simulink model "CAN_T_R_Model"  (R2018a)
settings: Solver=VariableStepAuto  StartTime=0.0  StopTime=10  RelTol=1e-3
undefined symbols (not defined in the file): canChannel
libraries: simulink x16, canlib x5, canmsglib x3
settings Model: Creator=arthu  LastModifiedBy=arthu

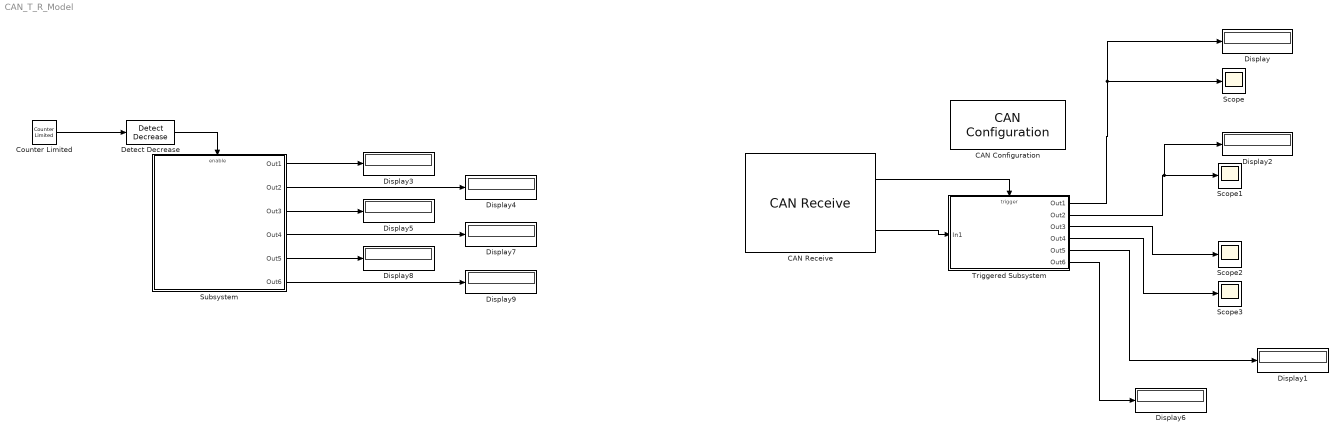
== system CAN_T_R_Model ==
  CAN Configuration : canlib/CAN Configuration  BlockHandle=2149.0007  DeviceMenu=(none)  Device=PEAK-System PCAN-USB (PCAN_USBBUS2)  ObjConstructor=canChannel('MathWorks','Virtual 1',1)  BusSpeed=1000000  EnableBitParameters=off  AckMode=Normal
      settings: SourceProductName=Vehicle Network Toolbox  SourceProductBaseCode=VN
  CAN Receive : canlib/CAN Receive  BlockHandle=2001.0005  DeviceMenu=(none)  Device=PEAK-System PCAN-USB (PCAN_USBBUS2)  ObjConstructor=canChannel('PEAK-System','PCAN_USBBUS1')  EnableStandardIDsFilter=off  StandardIDs=0  EnableExtendedIDsFilter=off  ExtendedIDs=0  SampleTime=0.001  MsgsPerTimestep=all  StdIDsCombo=Allow all  ExtIDsCombo=Allow all  InternalFilterUpdateStatus=on  BusOutput=off
      settings: SourceProductName=Vehicle Network Toolbox  SourceProductBaseCode=VN
  Counter Limited : simulink/Sources/Counter Limited  uplimit=24  tsamp=0.001
  Detect Decrease : simulink/Logic and Bit Operations/Detect Decrease  vinit=0.0  OutDataTypeStr=boolean
  Display{,1..9} (10 alike) : Display
  Scope{,1..3} (4 alike) : Scope
  Subsystem : Subsystem
  Triggered Subsystem : Subsystem  TreatAsAtomicUnit=on
  wires:
  Detect Decrease/1 -> Subsystem/Enable
  Counter Limited/1 -> Detect Decrease/1
  CAN Receive/2 -> Triggered Subsystem/1(In1)
  CAN Receive/1 -> Triggered Subsystem/Trigger
  Triggered Subsystem/1(Out1) -> Display/1, Scope/1
  Triggered Subsystem/2(Out2) -> Display2/1, Scope1/1
  Triggered Subsystem/3(Out3) -> Scope2/1
  Triggered Subsystem/4(Out4) -> Scope3/1
  Triggered Subsystem/5(Out5) -> Display1/1
  Subsystem/1(Out1) -> Display3/1
  Subsystem/2(Out2) -> Display4/1
  Subsystem/3(Out3) -> Display5/1
  Triggered Subsystem/6(Out6) -> Display6/1
  Subsystem/4(Out4) -> Display7/1
  Subsystem/6(Out6) -> Display9/1
  Subsystem/5(Out5) -> Display8/1

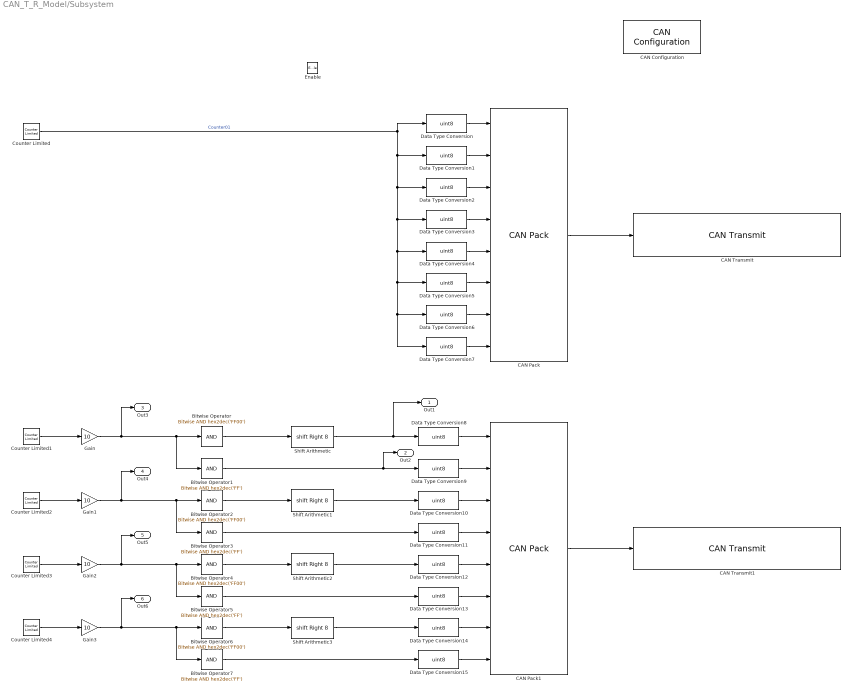
== system CAN_T_R_Model/Subsystem ==
  Enable : EnablePort
  Bitwise Operator{,2,4,6} (4 alike) : simulink/Logic and Bit Operations/Bitwise Operator  logicop=AND  UseBitMask=on  BitMask=hex2dec('FF00')  BitMaskRealWorld=Stored Integer
  Bitwise Operator{1,3,5,7} (4 alike) : simulink/Logic and Bit Operations/Bitwise Operator  logicop=AND  UseBitMask=on  BitMask=hex2dec('FF')  BitMaskRealWorld=Stored Integer
  CAN Configuration : canlib/CAN Configuration  BlockHandle=17.0002  DeviceMenu=PEAK-System PCAN-USB (PCAN_USBBUS1)  Device=PEAK-System PCAN-USB (PCAN_USBBUS1)  ObjConstructor=canChannel('PEAK-System','PCAN_USBBUS1')  BusSpeed=1000000  EnableBitParameters=off  AckMode=Normal
      settings: SourceProductName=Vehicle Network Toolbox  SourceProductBaseCode=VN
  CAN Pack : canmsglib/CAN Pack  MsgList=(none)  MsgName=CAN Msg  MsgIDType=Extended (29-bit identifier)  MsgIdentifier=2000  MsgLength=8  SignalInfo=Signal1$0$8$1$2$1$0$1$0$-Inf$Inf$#Signal2$8$8$1$2$1$0$1$0$-Inf$Inf$#Signal3$16$8$1$2$1$0$1$0$-Inf$Inf$#Signal4$24$8$1$2$1$0$1$0$-Inf$Inf$#Signal5$32$8$1$2$1$0$1$0$-Inf$Inf$#Signal6$40$8$1$2$1$0$1$0$-Inf$Inf$#Signal7$48$8$1$2$1$0$1$0$-Inf$Inf$#Signal8$56$8$1$2$1$0$1$0$-Inf$Inf$#  NSignals=8  StartBits=str2num('[int32(0);int32(8);int32(16);int32(24);int32(32);int32(40);int32(48);int32(56)]')  SignalSizes=str2num('[int32(8);int32(8);int32(8);int32(8);int32(8);int32(8);int32(8);int32(8)]')  ByteOrders=str2num('[int32(1);int32(1);int32(1);int32(1);int32(1);int32(1);int32(1);int32(1)]')  DataTypes=str2num('[int32(2);int32(2);int32(2);int32(2);int32(2);int32(2);int32(2);int32(2)]')  MultiplexTypes=str2num('[int32(1);int32(1);int32(1);int32(1);int32(1);int32(1);int32(1);int32(1)]')  MultiplexValues=str2num('[double(0);double(0);double(0);double(0);double(0);double(0);double(0);double(0)]')  Factors=str2num('[double(1);double(1);double(1);double(1);double(1);double(1);double(1);double(1)]')  Offsets=str2num('[double(0);double(0);double(0);double(0);double(0);double(0);double(0);double(0)]')  Minimums=str2num('[double(-Inf);double(-Inf);double(-Inf);double(-Inf);double(-Inf);double(-Inf);double(-Inf);double(-Inf)]')  Maximums=str2num('[double(Inf);double(Inf);double(Inf);double(Inf);double(Inf);double(Inf);double(Inf);double(Inf)]')  Remote=off  ApplyMinMax=off  BusOutput=off
      settings: SourceProductName=Simulink Real-Time  SourceProductBaseCode=XP  DataFormat=manually specified signals
  CAN Pack1 : canmsglib/CAN Pack  MsgList=(none)  MsgName=CAN Msg  MsgIDType=Extended (29-bit identifier)  MsgIdentifier=2001  MsgLength=8  SignalInfo=Signal1$0$8$1$2$1$0$1$0$-Inf$Inf$#Signal2$8$8$1$2$1$0$1$0$-Inf$Inf$#Signal3$16$8$1$2$1$0$1$0$-Inf$Inf$#Signal4$24$8$1$2$1$0$1$0$-Inf$Inf$#Signal5$32$8$1$2$1$0$1$0$-Inf$Inf$#Signal6$40$8$1$2$1$0$1$0$-Inf$Inf$#Signal7$48$8$1$2$1$0$1$0$-Inf$Inf$#Signal8$56$8$1$2$1$0$1$0$-Inf$Inf$#  NSignals=8  StartBits=str2num('[int32(0);int32(8);int32(16);int32(24);int32(32);int32(40);int32(48);int32(56)]')  SignalSizes=str2num('[int32(8);int32(8);int32(8);int32(8);int32(8);int32(8);int32(8);int32(8)]')  ByteOrders=str2num('[int32(1);int32(1);int32(1);int32(1);int32(1);int32(1);int32(1);int32(1)]')  DataTypes=str2num('[int32(2);int32(2);int32(2);int32(2);int32(2);int32(2);int32(2);int32(2)]')  MultiplexTypes=str2num('[int32(1);int32(1);int32(1);int32(1);int32(1);int32(1);int32(1);int32(1)]')  MultiplexValues=str2num('[double(0);double(0);double(0);double(0);double(0);double(0);double(0);double(0)]')  Factors=str2num('[double(1);double(1);double(1);double(1);double(1);double(1);double(1);double(1)]')  Offsets=str2num('[double(0);double(0);double(0);double(0);double(0);double(0);double(0);double(0)]')  Minimums=str2num('[double(-Inf);double(-Inf);double(-Inf);double(-Inf);double(-Inf);double(-Inf);double(-Inf);double(-Inf)]')  Maximums=str2num('[double(Inf);double(Inf);double(Inf);double(Inf);double(Inf);double(Inf);double(Inf);double(Inf)]')  Remote=off  ApplyMinMax=off  BusOutput=off
      settings: SourceProductName=Simulink Real-Time  SourceProductBaseCode=XP  DataFormat=manually specified signals
  CAN Transmit : canlib/CAN Transmit  BlockHandle=15.0001  DeviceMenu=PEAK-System PCAN-USB (PCAN_USBBUS1)  Device=PEAK-System PCAN-USB (PCAN_USBBUS1)  ObjConstructor=canChannel('PEAK-System','PCAN_USBBUS1')  EnablePeriodicTransmit=off  MessagePeriod=0.050
      settings: SourceProductName=Vehicle Network Toolbox  SourceProductBaseCode=VN
  CAN Transmit1 : canlib/CAN Transmit  BlockHandle=2090.0005  DeviceMenu=PEAK-System PCAN-USB (PCAN_USBBUS1)  Device=PEAK-System PCAN-USB (PCAN_USBBUS1)  ObjConstructor=canChannel('PEAK-System','PCAN_USBBUS1')  EnablePeriodicTransmit=off  MessagePeriod=0.050
      settings: SourceProductName=Vehicle Network Toolbox  SourceProductBaseCode=VN
  Counter Limited{,1..4} (5 alike) : simulink/Sources/Counter Limited  uplimit=255  tsamp=-1
  Data Type Conversion{,1..15} (16 alike) : DataTypeConversion  OutDataTypeStr=uint8
  Gain{,1..3} (4 alike) : Gain  Gain=10  OutDataTypeStr=uint16
  Shift Arithmetic{,1..3} (4 alike) : ArithShift  BitShiftNumber=8  BitShiftDirection=Right
  Out1 : Outport
  Out2 : Outport  Port=2
  Out3 : Outport  Port=3
  Out4 : Outport  Port=4
  Out5 : Outport  Port=5
  Out6 : Outport  Port=6
  wires:
  Data Type Conversion1/1 -> CAN Pack/2
  Data Type Conversion3/1 -> CAN Pack/4
  CAN Pack/1 -> CAN Transmit/1
  Data Type Conversion2/1 -> CAN Pack/3
  Data Type Conversion6/1 -> CAN Pack/7
  Data Type Conversion/1 -> CAN Pack/1
  Data Type Conversion5/1 -> CAN Pack/6
  Data Type Conversion7/1 -> CAN Pack/8
  Data Type Conversion4/1 -> CAN Pack/5
  CAN Pack1/1 -> CAN Transmit1/1
  Counter Limited/1 -> Data Type Conversion/1, Data Type Conversion6/1, Data Type Conversion7/1, Data Type Conversion5/1, Data Type Conversion4/1, Data Type Conversion3/1, Data Type Conversion2/1, Data Type Conversion1/1  "Counter01"
  Data Type Conversion8/1 -> CAN Pack1/1
  Data Type Conversion9/1 -> CAN Pack1/2
  Data Type Conversion10/1 -> CAN Pack1/3
  Data Type Conversion11/1 -> CAN Pack1/4
  Data Type Conversion12/1 -> CAN Pack1/5
  Data Type Conversion13/1 -> CAN Pack1/6
  Data Type Conversion14/1 -> CAN Pack1/7
  Data Type Conversion15/1 -> CAN Pack1/8
  Bitwise Operator/1 -> Shift Arithmetic/1
  Bitwise Operator1/1 -> Out2/1, Data Type Conversion9/1
  Shift Arithmetic/1 -> Out1/1, Data Type Conversion8/1
  Bitwise Operator3/1 -> Data Type Conversion11/1
  Bitwise Operator2/1 -> Shift Arithmetic1/1
  Shift Arithmetic1/1 -> Data Type Conversion10/1
  Bitwise Operator4/1 -> Shift Arithmetic2/1
  Bitwise Operator5/1 -> Data Type Conversion13/1
  Shift Arithmetic2/1 -> Data Type Conversion12/1
  Bitwise Operator7/1 -> Data Type Conversion15/1
  Bitwise Operator6/1 -> Shift Arithmetic3/1
  Shift Arithmetic3/1 -> Data Type Conversion14/1
  Counter Limited1/1 -> Gain/1
  Gain/1 -> Out3/1, Bitwise Operator1/1, Bitwise Operator/1
  Gain1/1 -> Bitwise Operator3/1, Bitwise Operator2/1, Out4/1
  Counter Limited2/1 -> Gain1/1
  Counter Limited3/1 -> Gain2/1
  Gain2/1 -> Out5/1, Bitwise Operator5/1, Bitwise Operator4/1
  Gain3/1 -> Bitwise Operator7/1, Bitwise Operator6/1, Out6/1
  Counter Limited4/1 -> Gain3/1

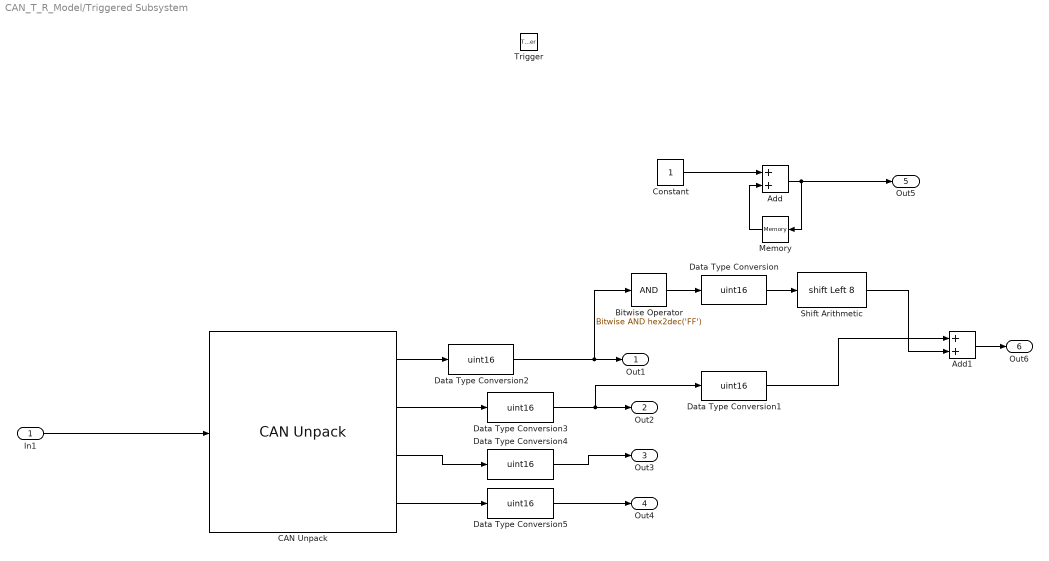
== system CAN_T_R_Model/Triggered Subsystem ==
  In1 : Inport
  Trigger : TriggerPort  TriggerType=function-call  VariantControl=Variant  PortDimensions=1
  Add : Sum
  Add1 : Sum
  Bitwise Operator : simulink/Logic and Bit Operations/Bitwise Operator  logicop=AND  UseBitMask=on  BitMask=hex2dec('FF')  BitMaskRealWorld=Stored Integer
  CAN Unpack : canmsglib/CAN Unpack  MsgList=(none)  MsgName=CAN Msg  MsgIDType=Extended (29-bit identifier)  MsgIdentifier=2001  MsgLength=8  SignalInfo=Signal1$0$8$1$2$1$0$1$0$-Inf$Inf$#Signal2$8$8$1$2$1$0$1$0$-Inf$Inf$#Signal3$16$8$1$2$1$0$1$0$-Inf$Inf$#Signal4$24$8$1$2$1$0$1$0$-Inf$Inf$#  NSignals=4  IDPort=off  TimestampPort=off  ErrorPort=off  RemotePort=off  LengthPort=off  StatusPort=off  StartBits=str2num('[int32(0);int32(8);int32(16);int32(24)]')  SignalSizes=str2num('[int32(8);int32(8);int32(8);int32(8)]')  ByteOrders=str2num('[int32(1);int32(1);int32(1);int32(1)]')  DataTypes=str2num('[int32(2);int32(2);int32(2);int32(2)]')  MultiplexTypes=str2num('[int32(1);int32(1);int32(1);int32(1)]')  MultiplexValues=str2num('[double(0);double(0);double(0);double(0)]')  Factors=str2num('[double(1);double(1);double(1);double(1)]')  Offsets=str2num('[double(0);double(0);double(0);double(0)]')  Minimums=str2num('[double(-Inf);double(-Inf);double(-Inf);double(-Inf)]')  Maximums=str2num('[double(Inf);double(Inf);double(Inf);double(Inf)]')  ApplyMinMax=off
      settings: SourceProductName=Simulink Real-Time  SourceProductBaseCode=XP
  Constant : Constant
  Data Type Conversion{,1..5} (6 alike) : DataTypeConversion  OutDataTypeStr=uint16
  Memory : Memory  InheritSampleTime=on
  Shift Arithmetic : ArithShift  BitShiftNumber=8  BitShiftDirection=Left
  Out1 : Outport
  Out2 : Outport  Port=2
  Out3 : Outport  Port=3
  Out4 : Outport  Port=4
  Out5 : Outport  Port=5
  Out6 : Outport  Port=6
  wires:
  In1/1 -> CAN Unpack/1
  CAN Unpack/1 -> Data Type Conversion2/1
  CAN Unpack/2 -> Data Type Conversion3/1
  CAN Unpack/3 -> Data Type Conversion4/1
  CAN Unpack/4 -> Data Type Conversion5/1
  Constant/1 -> Add/1
  Add/1 -> Out5/1, Memory/1
  Memory/1 -> Add/2
  Bitwise Operator/1 -> Data Type Conversion/1
  Data Type Conversion/1 -> Shift Arithmetic/1
  Shift Arithmetic/1 -> Add1/2
  Data Type Conversion1/1 -> Add1/1
  Add1/1 -> Out6/1
  Data Type Conversion2/1 -> Bitwise Operator/1, Out1/1
  Data Type Conversion3/1 -> Data Type Conversion1/1, Out2/1
  Data Type Conversion4/1 -> Out3/1
  Data Type Conversion5/1 -> Out4/1
